simulink model "preshaping"  (R2024b)
settings: Solver=VariableStepAuto  StartTime=0.0  StopTime=2  RelTol=1e-3
values from neighbouring files (symbols this model uses):
  a2 = shortened_step_value * 1/(1+K)    [simulate_preshaping.m]
  b2 = shortened_step_value    [simulate_preshaping.m]
  c2 = shortened_step_value * K/(1+K)    [simulate_preshaping.m]
  cruise_time = 1    [simulate_preshaping.m]
  deltaT = pi/(wn*sqrt(1-zeta^2))    [simulate_preshaping.m]
  initial_delay = 0.1    [simulate_preshaping.m]
  original_accel_time = 0.1    [simulate_preshaping.m]
  original_step_value = target_velocity / original_accel_time    (= 10)    [simulate_preshaping.m]
  shortened_step_time = original_accel_time - deltaT    [simulate_preshaping.m]
  wn = 100    [simulate_preshaping.m]
  zeta = 0.05    [simulate_preshaping.m]
settings Model: Creator=shohei  LastModifiedBy=shohei

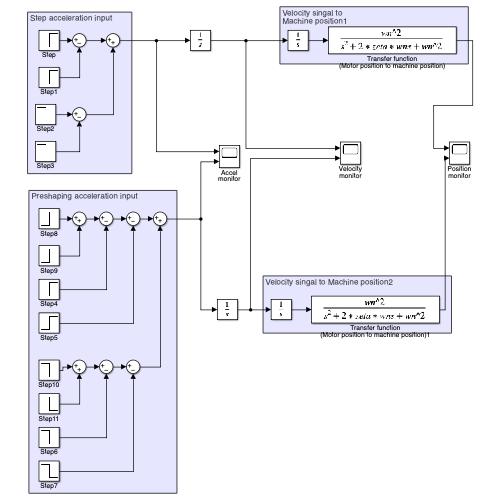
[thumbnail: Simulink's stored preview of the top-level diagram]
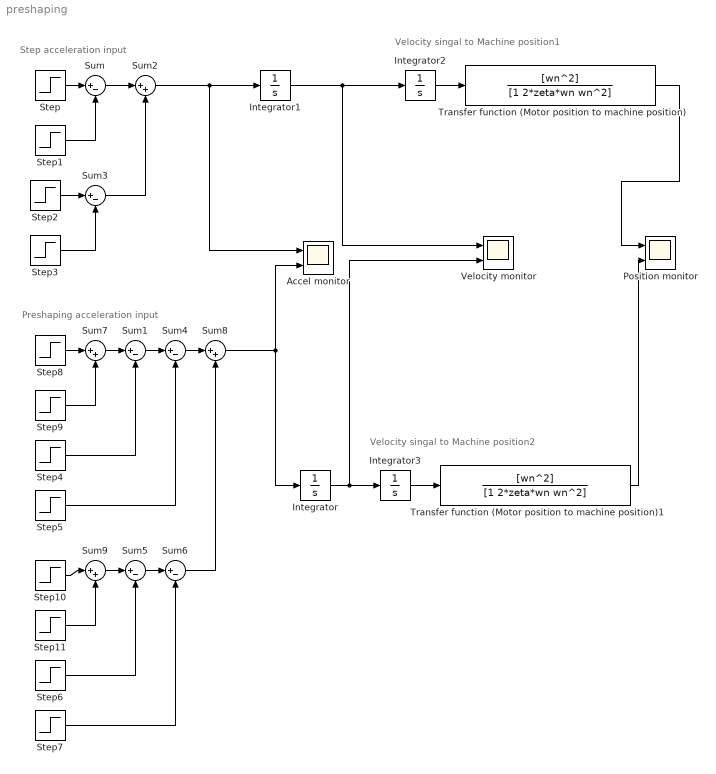
== system preshaping ==
  note: Preshaping acceleration input
  note: Velocity singal to Machine position2
  note: Velocity singal to
      | Machine position1
  note: Step acceleration input
  Accel monitor : Scope  NumInputPorts=2
  Integrator{,1..3} (4 alike) : Integrator
  Position monitor : Scope  NumInputPorts=2
  Step : Step  Time=initial_delay  After=original_step_value  SampleTime=0
  Step1 : Step  Time=initial_delay+original_accel_time  After=original_step_value  SampleTime=0
  Step10 : Step  Time=initial_delay+cruise_time  After=-a2  SampleTime=0
  Step11 : Step  Time=initial_delay++cruise_time+deltaT  After=-(b2-a2)  SampleTime=0
  Step2 : Step  Time=initial_delay+cruise_time  After=-original_step_value  SampleTime=0
  Step3 : Step  Time=initial_delay+cruise_time+original_accel_time  After=-original_step_value  SampleTime=0
  Step4 : Step  Time=initial_delay+shortened_step_time  After=a2  SampleTime=0
  Step5 : Step  Time=initial_delay+shortened_step_time+deltaT  After=c2  SampleTime=0
  Step6 : Step  Time=initial_delay++cruise_time+shortened_step_time  After=-a2  SampleTime=0
  Step7 : Step  Time=initial_delay++cruise_time+shortened_step_time+deltaT  After=-c2  SampleTime=0
  Step8 : Step  Time=initial_delay  After=a2  SampleTime=0
  Step9 : Step  Time=initial_delay+deltaT  After=b2-a2  SampleTime=0
  Sum{,1,3..6} (6 alike) : Sum  Inputs=|+-
  Sum{2,7..9} (4 alike) : Sum  Inputs=|++
  Transfer function (Motor position to machine position) : TransferFcn  Numerator=[wn^2]  Denominator=[1 2*zeta*wn wn^2]
  Transfer function (Motor position to machine position)1 : TransferFcn  Numerator=[wn^2]  Denominator=[1 2*zeta*wn wn^2]
  Velocity monitor : Scope  NumInputPorts=2
  wires:
  Sum8/1 -> Integrator/1, Accel monitor/2
  Sum2/1 -> Integrator1/1, Accel monitor/1
  Transfer function (Motor position to machine position)/1 -> Position monitor/1
  Transfer function (Motor position to machine position)1/1 -> Position monitor/2
  Step1/1 -> Sum/2
  Sum/1 -> Sum2/1
  Step3/1 -> Sum3/2
  Step/1 -> Sum/1
  Step2/1 -> Sum3/1
  Sum3/1 -> Sum2/2
  Integrator2/1 -> Transfer function (Motor position to machine position)/1
  Integrator1/1 -> Velocity monitor/1, Integrator2/1
  Integrator3/1 -> Transfer function (Motor position to machine position)1/1
  Integrator/1 -> Velocity monitor/2, Integrator3/1
  Step9/1 -> Sum7/2
  Sum7/1 -> Sum1/1
  Sum6/1 -> Sum8/2
  Step8/1 -> Sum7/1
  Sum9/1 -> Sum5/1
  Step10/1 -> Sum9/1
  Step5/1 -> Sum4/2
  Step6/1 -> Sum5/2
  Sum5/1 -> Sum6/1
  Step11/1 -> Sum9/2
  Sum1/1 -> Sum4/1
  Sum4/1 -> Sum8/1
  Step7/1 -> Sum6/2
  Step4/1 -> Sum1/2
